simulink model "vexv5_Clawbot_Auto_Stateflow"  (R2019a)
settings: Solver=ode3  StartTime=0.0  StopTime=inf  RelTol=1e-3  EnableMultiTasking=on
libraries: vexv5lib x4
settings Model: ExtModeTrigDuration=25  Creator=josea  LastModifiedBy=josea
settings DataIOCC: LimitDataPoints=on  SaveFormat=Array  ReturnWorkspaceOutputs=off
settings OptimizationCC: ExpressionDepthLimit=2147483647  LifeSpan=Inf  MaxStackSize=64
settings DebuggingCC: UnderspecifiedInitializationDetection=Classic  MergeDetectMultiDrivingBlocksExec=none  InheritedTsInSrcMsg=none  FcnCallInpInsideContextMsg=warning  UnconnectedInputMsg=none  UnconnectedOutputMsg=none  AllowSymbolicDim=off  StateNameClashWarn=warning  PregeneratedLibrarySubsystemCodeDiagnostic=none  SFUnexpectedBacktrackingDiag=warning  SFNoUnconditionalDefaultTransitionDiag=warning  SFExecutionAtInitializationDiag=none  ArithmeticOperatorsInVariantConditions=warning
settings HardwareCC: ProdBitPerPointer=32  ProdBitPerSizeT=32  ProdBitPerPtrDiffT=32  ProdLargestAtomicInteger=Long  ProdLargestAtomicFloat=Double  ProdWordSize=32  ProdHWDeviceType=ARM Compatible->ARM Cortex  UseEmbeddedCoderFeatures=off
settings ModelReferenceCC: PropagateSignalLabelsOutOfModel=off
settings SFSimCC: SimUseLocalCustomCode=off
settings RTWCC: SystemTargetFile=ert.tlc  HardwareBoard=VEX V5 Robot Brain  TLCOptions=-aInlineSetEventsForThisBaseRateFcn=TLC_FALSE -aSuppressMultiTaskScheduler=TLC_FALSE -aRateBasedStepFcn=0  TemplateMakefile=ert_default_tmf  RTWUseLocalCustomCode=off  Toolchain=GNU Tools for ARM Embedded Processors
settings CodeAppCC: StateflowObjectComments=on
settings ERTTargetCC: CodeReplacementLibrary=GCC ARM Cortex-M3  MultiwordLength=2048  ERTCustomFileBanners=off  SupportContinuousTime=on  SupportNonInlinedSFcns=on  RemoveResetFunc=off  ModelStepFunctionPrototypeControlCompliant=off  ConvertIfToSwitch=off  SuppressUnreachableDefaultCases=off
settings ConfigComp: CovMetricSettings=dw  CovHtmlReporting=on  CovSaveCumulativeToWorkspaceVar=on  CovSaveSingleToWorkspaceVar=on  CovExternalEMLEnable=off  CovSFcnEnable=off

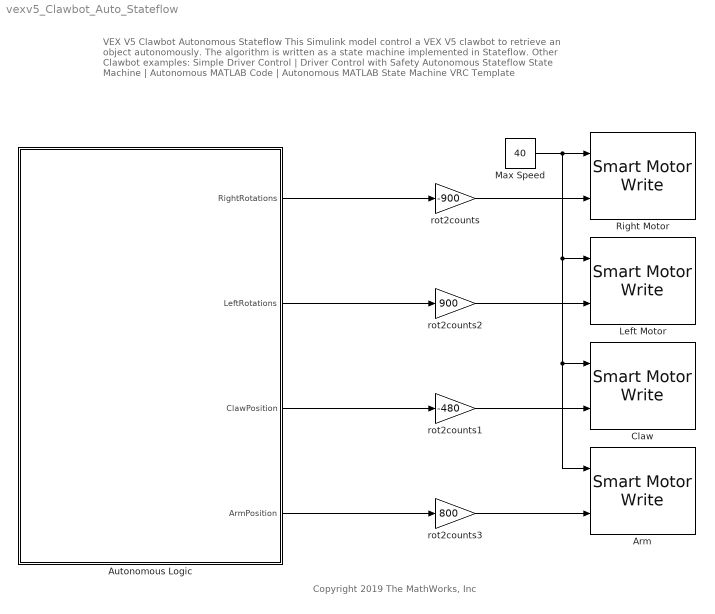
== system vexv5_Clawbot_Auto_Stateflow ==
  note: Copyright 2019 The MathWorks, Inc
  note: VEX V5 Clawbot Autonomous Stateflow
      | This Simulink model control a VEX V5 clawbot to retrieve an object autonomously.
      | The algorithm is written as a state machine implemented in Stateflow. Other Clawbot examples:
      | Simple Driver Control | Driver Control with Safety
      | Autonomous Stateflow State Machine | Autonomous MATLAB Code | Autonomous MATLAB State Machine
      | VRC Template
  Arm : vexv5lib/Actuators/Smart Motor Write  motorPort=8  scaleFactor=18:1  MotorBrakeMode=Hold  OperationMode=Position Control
      settings: SourceProductName=Simulink Coder Support Package for VEX EDR V5 Robot Brain
  Autonomous Logic : Stateflow chart  TreatAsAtomicUnit=on
  Claw : vexv5lib/Actuators/Smart Motor Write  motorPort=3  scaleFactor=18:1  MotorBrakeMode=Hold  OperationMode=Position Control
      settings: SourceProductName=Simulink Coder Support Package for VEX EDR V5 Robot Brain
  Left Motor : vexv5lib/Actuators/Smart Motor Write  motorPort=1  scaleFactor=18:1  MotorBrakeMode=Brake  OperationMode=Position Control
      settings: SourceProductName=Simulink Coder Support Package for VEX EDR V5 Robot Brain
  Max Speed : Constant  Value=40
  Right Motor : vexv5lib/Actuators/Smart Motor Write  motorPort=10  scaleFactor=18:1  MotorBrakeMode=Brake  OperationMode=Position Control
      settings: SourceProductName=Simulink Coder Support Package for VEX EDR V5 Robot Brain
  rot2counts : Gain  Gain=-900
  rot2counts1 : Gain  Gain=-480
  rot2counts2 : Gain  Gain=900
  rot2counts3 : Gain  Gain=800
  wires:
  Autonomous Logic/2(LeftRotations) -> rot2counts2/1
  rot2counts2/1 -> Left Motor/2
  Autonomous Logic/1(RightRotations) -> rot2counts/1
  rot2counts/1 -> Right Motor/2
  Autonomous Logic/3(ClawPosition) -> rot2counts1/1
  rot2counts1/1 -> Claw/2
  Max Speed/1 -> Claw/1, Arm/1, Left Motor/1, Right Motor/1
  Autonomous Logic/4(ArmPosition) -> rot2counts3/1
  rot2counts3/1 -> Arm/2

== stateflow chart vexv5_Clawbot_Auto_Stateflow/Autonomous Logic ==
  state MoveForward
    en:
    RightRotations=2;
    LeftRotations=2;
  state GrabObject
    en:
    ClawPosition=0;
  state LiftObject
    en:
    ArmPosition=1;
  state TurnAround
    en:
    RightRotations=RightRotations+1.5;
    LeftRotations=LeftRotations-1.5;
  state MoveBackward
    en:
    RightRotations=RightRotations+2;
    LeftRotations=LeftRotations+2;
  state DropObject
    en:
    ArmPosition=0;
    ClawPosition=1;
  (default) -> MoveForward : {ClawPosition=1;
      | ArmPosition=0;}
  MoveForward -> GrabObject : after(4,sec)
  GrabObject -> LiftObject : after(0.5,sec)
  LiftObject -> TurnAround : after(0.5,sec)
  TurnAround -> MoveBackward : after(4,sec)
  MoveBackward -> DropObject : after(4,sec)
  data: RightRotations output; LeftRotations output; ClawPosition output; ArmPosition output
